simulink model "comp_offset_input"  (R2018b)
settings: Solver=VariableStepAuto  StartTime=0.0  StopTime=10.0  RelTol=1e-3
libraries: simulink x1
settings Model: Creator=iamcy  LastModifiedBy=iamcy

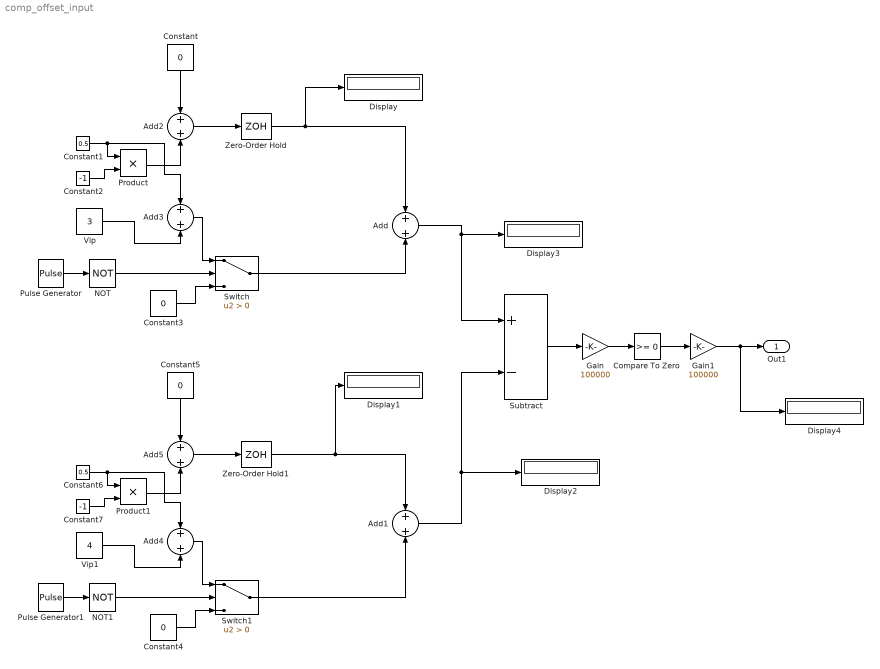
== system comp_offset_input ==
  Add{,1..5} (6 alike) : Sum  Inputs=2
  Compare To Zero : simulink/Logic and Bit Operations/Compare To Zero  relop=>=  OutDataTypeStr=boolean
  Constant{,3..5} (4 alike) : Constant  Value=0
  Constant1 : Constant  Value=0.5
  Constant2 : Constant  Value=-1
  Constant6 : Constant  Value=0.5
  Constant7 : Constant  Value=-1
  Display{,1..4} (5 alike) : Display
  Gain : Gain  Gain=100000
  Gain1 : Gain  Gain=100000
  NOT : Logic  Operator=NOT  IconShape=distinctive  AllPortsSameDT=off  OutDataTypeStr=boolean
  NOT1 : Logic  Operator=NOT  IconShape=distinctive  AllPortsSameDT=off  OutDataTypeStr=boolean
  Product : Product
  Product1 : Product
  Pulse Generator : DiscretePulseGenerator  PulseType=Time based  Period=13  PulseWidth=100/13
  Pulse Generator1 : DiscretePulseGenerator  PulseType=Time based  Period=13  PulseWidth=100/13
  Subtract : Sum  Inputs=+-
  Switch : Switch  Criteria=u2 > Threshold
  Switch1 : Switch  Criteria=u2 > Threshold
  Vip : Constant  Value=3
  Vip1 : Constant  Value=4
  Zero-Order Hold : ZeroOrderHold  SampleTime=-1
  Zero-Order Hold1 : ZeroOrderHold  SampleTime=-1
  Out1 : Outport
  wires:
  Subtract/1 -> Gain/1
  Gain1/1 -> Display4/1, Out1/1
  Compare To Zero/1 -> Gain1/1
  Gain/1 -> Compare To Zero/1
  Add/1 -> Subtract/1, Display3/1
  Add1/1 -> Subtract/2, Display2/1
  Zero-Order Hold/1 -> Display/1, Add/1
  Add2/1 -> Zero-Order Hold/1
  Constant/1 -> Add2/1
  Pulse Generator/1 -> NOT/1
  NOT/1 -> Switch/2
  Constant1/1 -> Add3/1, Product/1
  Constant2/1 -> Product/2
  Product/1 -> Add2/2
  Vip/1 -> Add3/2
  Add3/1 -> Switch/1
  Constant3/1 -> Switch/3
  Switch/1 -> Add/2
  Pulse Generator1/1 -> NOT1/1
  NOT1/1 -> Switch1/2
  Constant4/1 -> Switch1/3
  Add4/1 -> Switch1/1
  Vip1/1 -> Add4/2
  Switch1/1 -> Add1/2
  Product1/1 -> Add5/2
  Add5/1 -> Zero-Order Hold1/1
  Constant5/1 -> Add5/1
  Constant7/1 -> Product1/2
  Constant6/1 -> Add4/1, Product1/1
  Zero-Order Hold1/1 -> Display1/1, Add1/1
